simulink model "model_task3"  (R2022b)
settings: Solver=VariableStepAuto  StartTime=0.0  StopTime=10.0  RelTol=1e-3
settings Model: Creator=anton  LastModifiedBy=anton

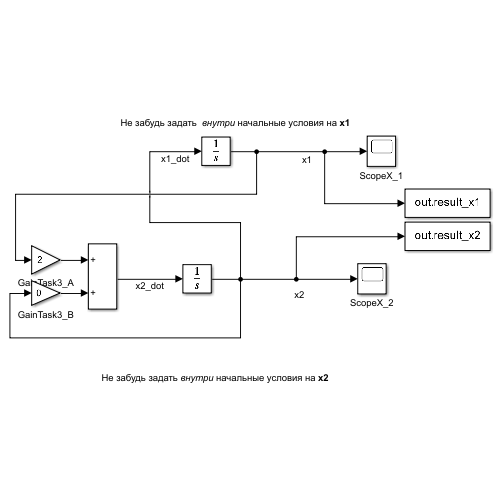
[thumbnail: Simulink's stored preview of the top-level diagram]
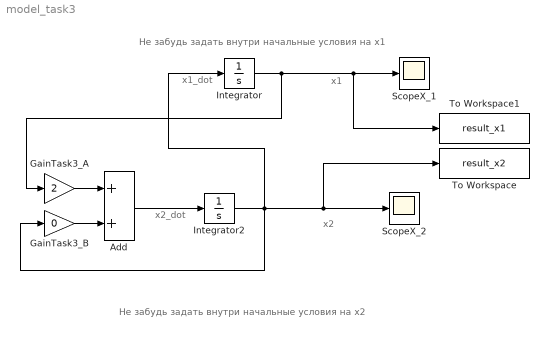
== system model_task3 ==
  note: Не забудь задать внутри начальные условия на x2
  note: Не забудь задать внутри начальные условия на x1
  note: x2_dot
  note: x1_dot
  note: x1
  note: x2
  Add : Sum
  GainTask3_A : Gain  Gain=2
  GainTask3_B : Gain  Gain=0
  Integrator : Integrator  InitialCondition=-1
  Integrator2 : Integrator  InitialCondition=-1
  ScopeX_1 : Scope
  ScopeX_2 : Scope
  To Workspace : ToWorkspace  VariableName=result_x2  SaveFormat=Timeseries  SampleTime=-1
  To Workspace1 : ToWorkspace  VariableName=result_x1  SaveFormat=Timeseries  SampleTime=-1
  wires:
  Integrator/1 -> GainTask3_A/1, To Workspace1/1, ScopeX_1/1
  Integrator2/1 -> GainTask3_B/1, To Workspace/1, ScopeX_2/1, Integrator/1
  Add/1 -> Integrator2/1
  GainTask3_B/1 -> Add/2
  GainTask3_A/1 -> Add/1
